simulink model "Final_Project_Part_2_Template"  (R2022a)
settings: Solver=FixedStepAuto  StartTime=0.0  StopTime=tspan  FixedStep=10  RelTol=1e-3
values from neighbouring files (symbols this model uses):
  E_b_ECI_0 = C2EulerAngles(C_b_ECI_0)    [Final_Project_Part_2_init_Template.m]
  q_b_ECI_0 = C2quat(C_b_ECI_0)    [Final_Project_Part_2_init_Template.m]
  T = [0;0;0]    [Final_Project_Part_2_init_Template.m]
  w_b_ECI_0 = [0.001; -0.001; 0.002]    [Final_Project_Part_2_init_Template.m]
undefined symbols (not defined in the file or in its folder): J
settings Model: Creator=emehiel  LastModifiedBy=emehiel
settings SolverCC: AlgebraicLoopSolver=TrustRegion
settings DebuggingCC: UnconnectedInputMsg=warning  UnconnectedOutputMsg=warning  UnconnectedLineMsg=warning  SFMachineParentedDataDiag=warning

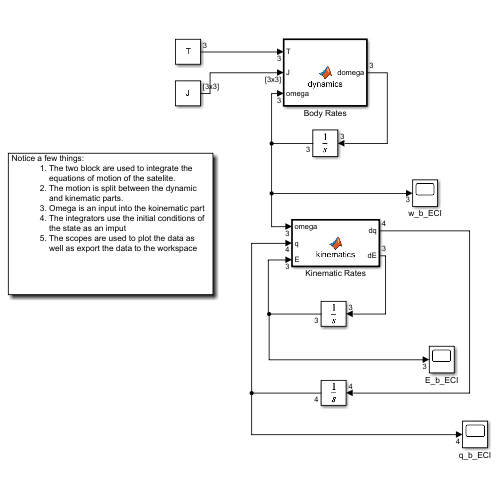
[thumbnail: Simulink's stored preview of the top-level diagram]
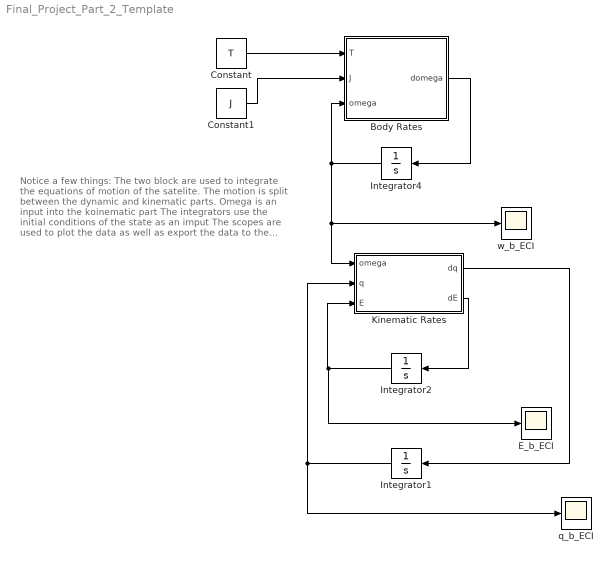
== system Final_Project_Part_2_Template ==
  note: Notice a few things:
      | The two block are used to integrate the equations of motion of the satelite.
      | The motion is split between the dynamic and kinematic parts.
      | Omega is an input into the koinematic part
      | The integrators use the initial conditions of the state as an imput
      | The scopes are used to plot the data as well as export the data to the workspace
  Body Rates : MATLAB Function  TreatAsAtomicUnit=on
  Constant : Constant  Value=T
  Constant1 : Constant  Value=J
  E_b_ECI : Scope
  Integrator1 : Integrator  InitialCondition=q_b_ECI_0
  Integrator2 : Integrator  InitialCondition=E_b_ECI_0
  Integrator4 : Integrator  InitialCondition=w_b_ECI_0
  Kinematic Rates : MATLAB Function  TreatAsAtomicUnit=on
  q_b_ECI : Scope
  w_b_ECI : Scope
  wires:
  Constant/1 -> Body Rates/1(T)
  Constant1/1 -> Body Rates/2(J)
  Body Rates/1(domega) -> Integrator4/1
  Integrator4/1 -> Body Rates/3(omega), w_b_ECI/1, Kinematic Rates/1(omega)
  Integrator2/1 -> E_b_ECI/1, Kinematic Rates/3(E)
  Integrator1/1 -> q_b_ECI/1, Kinematic Rates/2(q)
  Kinematic Rates/2(dE) -> Integrator2/1
  Kinematic Rates/1(dq) -> Integrator1/1

== matlab function Final_Project_Part_2_Template/Kinematic Rates ==
  data: omega input; q input; dq output; E input; dE output
function [dq,dE] = kinematics(omega, q, E)
%#codegen

% unpack quaternion

% compute the derivative of the quaternion components here

% compute the derivative of the Euler Angle components here

== matlab function Final_Project_Part_2_Template/Body Rates ==
  data: T input; J input; omega input; domega output
function domega = dynamics(T, J, omega)
%#codegen

% Compute the derivative of the angular velocity $\omega$ here
